simulink model "system_id_SOFCI_CL_test"  (R2022b)
settings: Solver=FixedStepAuto  StartTime=0.0  StopTime=time_final  RelTol=1e-3  EnableMultiTasking=on
values from neighbouring files (symbols this model uses):
  K_aug = [K_SF,K_int]    [step_response_our_repff.m]    (also in system_id_CLSOFCI.m; system_id_SOFCI_CL.m)
  signal_num = 1    [system_id_SOFCI_CL.m]
  Stepsize = 0.5    [step_response_our_repff.m]    (also in system_id_CLSOFCI.m = 0.4; system_id_SOFCI_CL.m = 0.4)
  time_final = 20    [system_id_CLSOFCI.m]    (also in system_id_SOFCI_CL.m)
  time_step = 10    [system_id_CLSOFCI.m]    (also in system_id_SOFCI_CL.m)
  Ts = 0.001    [step_response_our_repff.m]    (also in system_id_CLSOFCI.m; system_id_SOFCI_CL.m = TS(2))
  unit_period = 1    [system_id_SOFCI_CL.m]
undefined symbols (not defined in the file or in its folder): A_d, Ad, B_d, Bd, C_d, L_Pred, N
libraries: simulink x1
settings Model: ExtModeTrigDuration=8  Creator=Alex Zhen  LastModifiedBy=Alex Zhen
settings OptimizationCC: DefaultUnderspecifiedDataType=single  EnhancedBackFolding=on  PassReuseOutputArgsAs=Individual arguments  MaxStackSize=1024  OptimizeBlockOrder=speed  DifferentSizesBufferReuse=on  OptimizationCustomize=off  DenormalBehavior=FlushToZero  EfficientTunableParamExpr=on
settings DebuggingCC: ParameterTunabilityLossMsg=error
settings HardwareCC: ProdBitPerChar=16  ProdBitPerInt=16  ProdBitPerPointer=32  ProdBitPerSizeT=32  ProdBitPerPtrDiffT=32  ProdLargestAtomicInteger=Integer  ProdLargestAtomicFloat=None  ProdWordSize=16  ProdLongLongMode=on  ProdHWDeviceType=Texas Instruments->C2000
settings SFSimCC: MATLABDynamicMemAlloc=off
settings RTWCC: Description=Embedded Coder  SystemTargetFile=ert.tlc  HardwareBoard=TI Delfino F28379D LaunchPad  TLCOptions=-aInlineSetEventsForThisBaseRateFcn=TLC_FALSE -aSuppressMultiTaskScheduler=TLC_FALSE -aRateBasedStepFcn=1  TemplateMakefile=ert_default_tmf  Toolchain=Texas Instruments Code Composer Studio (C2000)
settings CodeAppCC: ForceParamTrailComments=on  IgnoreCustomStorageClasses=off  OperatorAnnotations=on  SimulinkDataObjDesc=on  SFDataObjDesc=on  InsertBlockDesc=on
settings ERTTargetCC: CodeReplacementLibrary=TI C28x  SupportContinuousTime=on  ExtModeTransport=4  ExtModeStaticAlloc=on  ExtModeAutomaticAllocSize=off  ExtModeMexFile=ext_xcp  ExtModeIntrfLevel=Level2 - Open

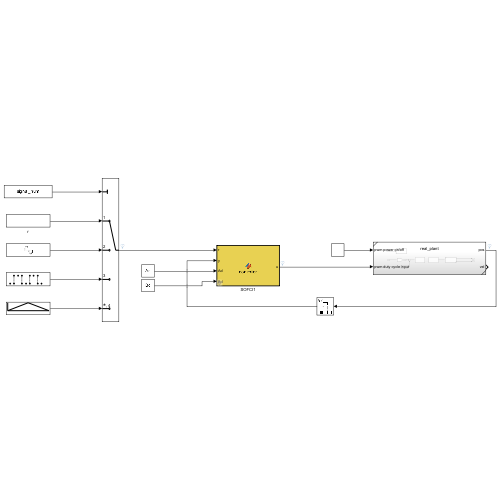
[thumbnail: Simulink's stored preview of the top-level diagram]
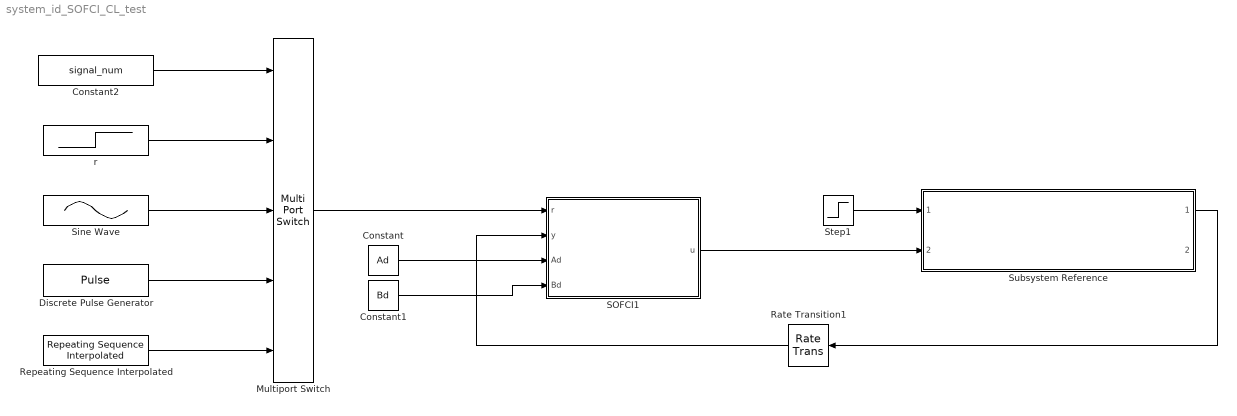
== system system_id_SOFCI_CL_test ==
  Constant : Constant  Value=Ad
  Constant1 : Constant  Value=Bd
  Constant2 : Constant  Value=signal_num
  Discrete Pulse Generator : DiscretePulseGenerator  Amplitude=Stepsize  Period=1/Ts  PulseWidth=1/Ts/2  SampleTime=Ts
  Multiport Switch : MultiPortSwitch  Inputs=4  SaturateOnIntegerOverflow=off  InputSameDT=off
  Rate Transition1 : RateTransition  Deterministic=off  OutPortSampleTime=Ts
  Repeating Sequence Interpolated : simulink/Sources/Repeating Sequence Interpolated  OutValues=[0 Stepsize 0]  TimeValues=[0 unit_period/2 unit_period]  LookUpMeth=Interpolation-Use End Values  tsamp=Ts  OutMin=[]  OutMax=[]  OutDataTypeStr=double  OutputDataTypeScalingMode=double  OutDataType=fixdt(0,8)  OutScaling=2^-10
  SOFCI1 : MATLAB Function  TreatAsAtomicUnit=on  mask{A=A_d, B=B_d, C=C_d, K=K_aug, L=L_Pred, N=N}
  Sine Wave : Sin  Amplitude=Stepsize/2  Bias=Stepsize/2  Frequency=2*pi/(1/unit_period)  SampleTime=Ts
  Step1 : Step  Time=time_final  Before=1  After=0  SampleTime=0
  Subsystem Reference : Subsystem  ReferencedSubsystem=real_plant
  r : Step  Time=time_step  After=Stepsize  SampleTime=Ts
  wires:
  Subsystem Reference/1 -> Rate Transition1/1
  Step1/1 -> Subsystem Reference/1
  Rate Transition1/1 -> SOFCI1/2(y)
  r/1 -> Multiport Switch/2
  SOFCI1/1(u) -> Subsystem Reference/2
  Constant/1 -> SOFCI1/3(Ad)
  Constant1/1 -> SOFCI1/4(Bd)
  Discrete Pulse Generator/1 -> Multiport Switch/4
  Repeating Sequence Interpolated/1 -> Multiport Switch/5
  Constant2/1 -> Multiport Switch/1
  Sine Wave/1 -> Multiport Switch/3
  Multiport Switch/1 -> SOFCI1/1(r)

== matlab function system_id_SOFCI_CL_test/SOFCI1 ==
  data: r input; u output; y input; A parameter; B parameter; C parameter; K parameter; L parameter; N parameter; Ad input; Bd input
function u = controller(r,y,A, B, C, K, L, N,Ad,Bd)

persistent xhat xint;  %memory for the state

  if isempty(xhat)  %local variable initialization
      n=size(L,1);
        xhat=zeros(n,1); 
      m = size(K,2)-n;
        xint=zeros(m,1);  
  end
xaug=[xhat; xint]; %Augmented state include the state for the integrator
%u = -K*xaug+N*r; %Control computation with integral action 
u_unsat = -K*xaug+N*r; %Control computation with integral action 
u= sign(u_unsat)*min(1,abs(u_unsat));
%DAC(u) send out control here to minimize computation delay
%Update the next state next
xhat = (A-L*C)*xhat + B*u + L*y;
xint = Ad * xint+ Bd * (y-r);
